simulink model "practice1"  (R2016a)
settings: Solver=VariableStepAuto  StartTime=0.0  StopTime=10.0  RelTol=1e-3
undefined symbols (not defined in the file or in its folder): Rec, SDTV
libraries: visionconversions x2, visionsources x2
settings Model: Creator=Auroshis  LastModifiedBy=Auroshis

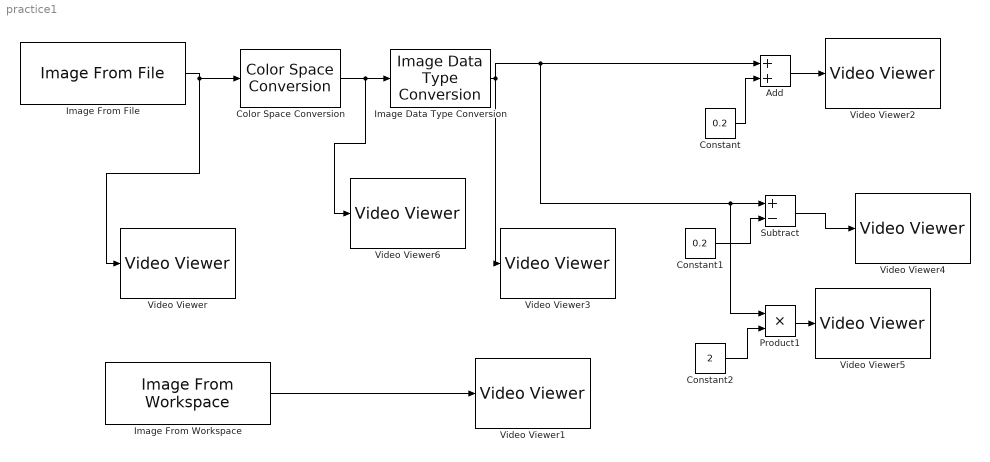
== system practice1 ==
  Add : Sum
  Color Space Conversion : visionconversions/Color Space  Conversion  conversion=Obsolete  conversionActive=R'G'B' to intensity  wp_str=D65  rec=Rec. 601 (SDTV)  sys=1125/60/2:1  imagePorts=One multidimensional signal
  Constant : Constant  Value=0.2  SampleTime=0.1
  Constant1 : Constant  Value=0.2  SampleTime=0.1
  Constant2 : Constant  Value=2  SampleTime=0.1
  Image Data Type Conversion : visionconversions/Image Data Type Conversion  outDT=double  isSigned=on  wordLen=16  numFracBits=0
  Image From File : visionsources/Image From File  Tag=vipblks_nd  FileName=peppers.png  imagePorts=One multidimensional signal  Ts=1  ImageDataType=Inherit from input image  Signed=on  WordLength=16  sdImageDataType=uint(8)  FractionLengthMode=User-defined  FractionLength=15  OutPortLabels=R|G|B
  Image From Workspace : visionsources/Image From Workspace  Tag=vipblks_nd  ImageValue=temp1  Ts=1  imagePorts=One multidimensional signal  ImageDataType=Inherit from 'Value'  Signed=on  WordLength=16  sdImageDataType=sfix(16)  FractionLengthMode=User-defined  FractionLength=15  OutPortLabels=R|G|B
  Product1 : Product
  Subtract : Sum  Inputs=+-
  Video Viewer : VideoViewer  FigPos=[1 822 1536 724]
  Video Viewer1 : VideoViewer  FigPos=[1068.2 499.6 409.6 300]
  Video Viewer2 : VideoViewer  Tag=addition
  Video Viewer3 : VideoViewer
  Video Viewer4 : VideoViewer  FigPos=[261.8 810 409.6 300]
  Video Viewer5 : VideoViewer  FigPos=[201.8 482.8 409.6 300]
  Video Viewer6 : VideoViewer
  wires:
  Image From File/1 -> Color Space Conversion/1, Video Viewer/1
  Image From Workspace/1 -> Video Viewer1/1
  Color Space Conversion/1 -> Video Viewer6/1, Image Data Type Conversion/1
  Image Data Type Conversion/1 -> Video Viewer3/1, Product1/1, Subtract/1, Add/1
  Constant/1 -> Add/2
  Constant1/1 -> Subtract/2
  Constant2/1 -> Product1/2
  Add/1 -> Video Viewer2/1
  Subtract/1 -> Video Viewer4/1
  Product1/1 -> Video Viewer5/1
